simulink model "quad_sim"  (Simulink 6.2)
settings: Solver=ode45  StartTime=0.0  StopTime=70  MaxStep=0.001  RelTol=1e-3
libraries: aerospace x2

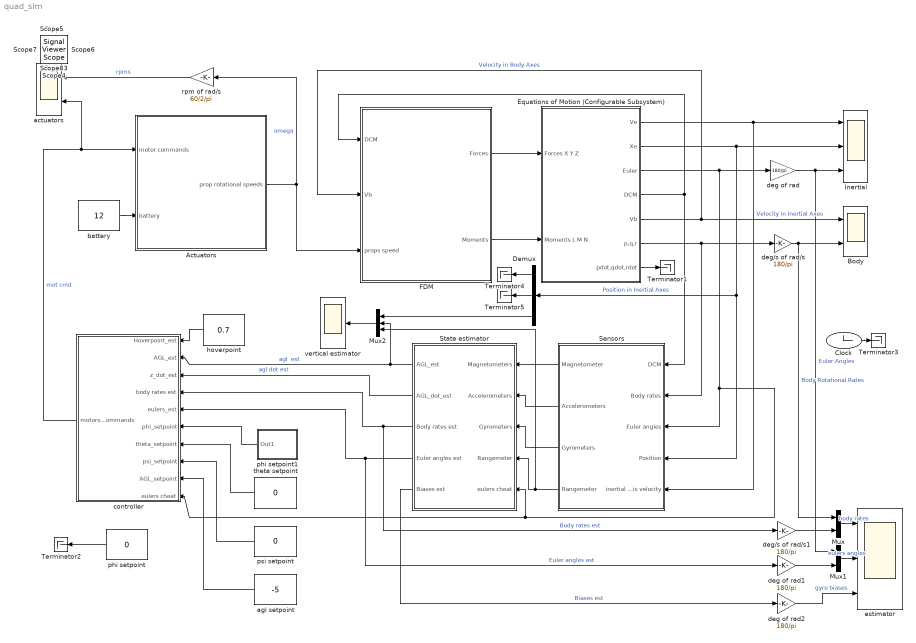
== system quad_sim ==
  Actuators : Subsystem  mask{Kv=1500, Tau=25, Kq=0.02}
  Body : Scope  NumInputPorts=2
  Clock : Clock
  Demux : Demux  Orientation=left  Outputs=3
  Equations of Motion (Configurable Subsystem) : Subsystem  BlockChoice=Euler Angles
      link override Euler Angles: Mass=0.5  Vm_0=[0 0 0]  Inertia=[0.0112 0 0; 0 0.0112 0; 0 0 0.0225]
  FDM : Subsystem  mask{Rho=1.225, Prop_area=0.005, Prop_radius=0.125, Mass=0.5, L=0.25, Ct=1.05, Cq=1.0, Cd_b=0.15}
      mask prompts: L "arm len"; Ct "Thrust aerodynamic coef"; Cq "Moment aerodynamic coef"; Cd_b "Body drag coef"
  Inertial : Scope  NumInputPorts=3
  Mux : Mux  Inputs=2
  Mux1 : Mux  Inputs=2
  Mux2 : Mux  Orientation=left  Inputs=3
  Sensors : Subsystem  Orientation=left
  State estimator : Subsystem  Orientation=left
  Terminator{1..5} (5 alike) : Terminator
  actuators : Scope  NumInputPorts=2
  agl setpoint : Constant  Orientation=left  Value=-5
  battery : Constant  Value=12
  controller : Subsystem  Orientation=left  mask{Kp_z=0.2, Kd_z=0.2, Kp_phi=-1.5, Kd_phi=-2.5, Kp_psi=-0.5, Kd_psi=-0.5}
  deg of rad : Gain  Gain=180/pi  SaturateOnIntegerOverflow=on
  deg of rad1 : Gain  Gain=180/pi  SaturateOnIntegerOverflow=on
  deg of rad2 : Gain  Gain=180/pi  SaturateOnIntegerOverflow=on
  deg/s of rad/s : Gain  Gain=180/pi  SaturateOnIntegerOverflow=on
  deg/s of rad/s1 : Gain  Gain=180/pi  SaturateOnIntegerOverflow=on
  estimator : Scope  NumInputPorts=3
  hoverpoint : Constant  Orientation=left  Value=0.7
  phi setpoint : Constant  Orientation=left  Value=0
  phi setpoint1 : Subsystem  Orientation=left  mask(timed input){t=[0 10 10 20 20 30 30 40 40 60], u=[0 0  -1 -1 0 0 1 1 0 0]*10/180*pi}
      mask prompts: t "time values:"; u "input values"
  psi setpoint : Constant  Orientation=left  Value=0
  rpm of rad/s : Gain  Orientation=left  Gain=60/2/pi  SaturateOnIntegerOverflow=on
  theta setpoint : Constant  Orientation=left  Value=0
  vertical estimator : Scope
  Scope{,1..8} (9 alike) : SignalViewerScope  IOType=viewer  RefreshTime=0.035000
  wires:
  Clock/1 -> Terminator3/1
  Equations of Motion (Configurable Subsystem)/3(Euler) -> deg of rad/1, Sensors/3(Euler angles), State estimator/5(eulers cheat), controller/10(eulers cheat)
  Equations of Motion (Configurable Subsystem)/5(Vb) -> Body/1, FDM/2(Vb)  "Velocity in Body Axes"
  Equations of Motion (Configurable Subsystem)/1(Ve) -> Inertial/1, Sensors/5(inertial axis velocity)  "Velocity in Inertial Axes"
  Equations of Motion (Configurable Subsystem)/2(Xe) -> Inertial/2, Sensors/4(Position), Demux/1  "Position in Inertial Axes"
  deg of rad/1 -> Inertial/3, Mux1/1  "Euler Angles"
  Equations of Motion (Configurable Subsystem)/6(p,q,r) -> deg/s of rad/s/1, Sensors/2(Body rates)
  deg/s of rad/s/1 -> Body/2, Mux/1  "Body Rotational Rates"
  Equations of Motion (Configurable Subsystem)/7(pdot,qdot,rdot) -> Terminator1/1
  FDM/2(Moments) -> Equations of Motion (Configurable Subsystem)/2(Moments L M N)
  FDM/1(Forces) -> Equations of Motion (Configurable Subsystem)/1(Forces X Y Z)
  Equations of Motion (Configurable Subsystem)/4(DCM) -> FDM/1(DCM), Sensors/1(DCM)
  battery/1 -> Actuators/2(battery)
  Actuators/1(prop rotational speeds) -> rpm of rad/s/1, FDM/3(props speed)  "omega"
  rpm of rad/s/1 -> actuators/1  "rpms"
  controller/1(motors commands) -> Actuators/1(motor commands), actuators/2  "mot cmd"
  hoverpoint/1 -> controller/1(Hoverpoint_est)
  agl setpoint/1 -> controller/9(AGL_setpoint)
  Sensors/4(Rangemeter) -> State estimator/4(Rangemeter), Mux2/3
  psi setpoint/1 -> controller/8(psi_setpoint)
  theta setpoint/1 -> controller/7(theta_setpoint)
  State estimator/3(Body rates est) -> controller/4(body rates est), deg/s of rad/s1/1  "Body rates est"
  State estimator/4(Euler angles est) -> controller/5(eulers_est), deg of rad1/1  "Euler angles est"
  Sensors/1(Magnetometer) -> State estimator/1(Magnetometers)
  Sensors/2(Accelerometers) -> State estimator/2(Accelerometers)
  Sensors/3(Gyrometers) -> State estimator/3(Gyrometers)
  Mux/1 -> estimator/1  "body rates"
  deg/s of rad/s1/1 -> Mux/2
  Mux1/1 -> estimator/2  "eulers angles"
  deg of rad1/1 -> Mux1/2
  phi setpoint1/1(Out1) -> controller/6(phi_setpoint)
  deg of rad2/1 -> estimator/3  "gyro biases"
  State estimator/5(Biases est) -> deg of rad2/1  "Biases est"
  phi setpoint/1 -> Terminator2/1
  Mux2/1 -> vertical estimator/1
  Demux/1 -> Terminator4/1
  Demux/2 -> Terminator5/1
  Demux/3 -> Mux2/1
  State estimator/1(AGL_est) -> controller/2(AGL_est), Mux2/2  "agl  est"
  State estimator/2(AGL_dot_est) -> controller/3(z_dot_est)  "agl dot est"

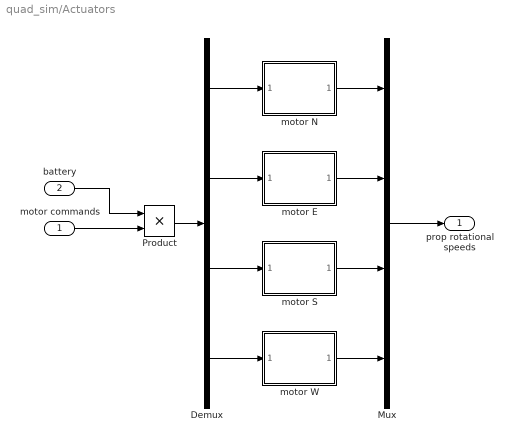
== system quad_sim/Actuators ==
  motor commands : Inport  Port=1  LatchInput=off
  battery : Inport  Port=2  LatchInput=off
  Demux : Demux
  Mux : Mux
  Product : Product  RndMeth=Zero
  motor E : Subsystem
  motor N : Subsystem
  motor S : Subsystem
  motor W : Subsystem
  prop rotational speeds : Outport
  wires:
  motor commands/1 -> Product/2
  battery/1 -> Product/1
  Product/1 -> Demux/1
  Mux/1 -> prop rotational speeds/1
  Demux/1 -> motor N/1(voltage)
  Demux/2 -> motor E/1(voltage)
  Demux/3 -> motor S/1(voltage)
  Demux/4 -> motor W/1(voltage)
  motor N/1(omega) -> Mux/1
  motor E/1(omega) -> Mux/2
  motor S/1(omega) -> Mux/3
  motor W/1(omega) -> Mux/4

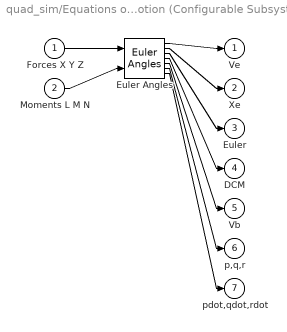
== system quad_sim/Equations of Motion (Configurable Subsystem) ==
  Forces X Y Z : Inport  Port=1  LatchInput=off
  Moments L M N : Inport  Port=2  LatchInput=off
  Euler Angles : aerospace/6DoF/Euler Angles  xme_0=[0 0 0]  Vm_0=[0 0 0]  eul_0=[0 0 0]  pm_0=[0 0 0]  Mass=0.5  Inertia=[0.0112 0 0; 0 0.0112 0; 0 0 0.0225]
  Ve : Outport
  Xe : Outport  Port=2
  Euler : Outport  Port=3
  DCM : Outport  Port=4
  Vb : Outport  Port=5
  p,q,r : Outport  Port=6
  pdot,qdot,rdot : Outport  Port=7
  wires:
  Forces X Y Z/1 -> Euler Angles/1
  Moments L M N/1 -> Euler Angles/2
  Euler Angles/1 -> Ve/1
  Euler Angles/2 -> Xe/1
  Euler Angles/3 -> Euler/1
  Euler Angles/4 -> DCM/1
  Euler Angles/5 -> Vb/1
  Euler Angles/6 -> p,q,r/1
  Euler Angles/7 -> pdot,qdot,rdot/1

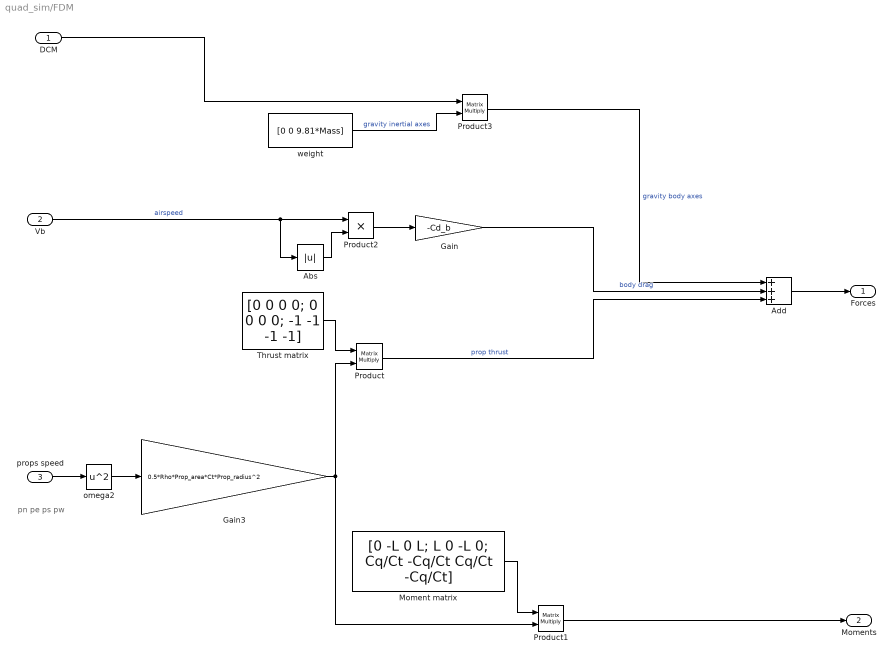
== system quad_sim/FDM ==
  note: pn
      | pe
      | ps
      | pw
  DCM : Inport  Port=1  LatchInput=off
  Vb : Inport  Port=2  LatchInput=off
  props speed : Inport  Port=3  LatchInput=off
  Abs : Abs
  Add : Sum  Inputs=+++  OutScaling=2^-10
  Gain : Gain  Gain=-Cd_b
  Gain3 : Gain  Gain=0.5*Rho*Prop_area*Ct*Prop_radius^2
  Moment matrix : Constant  Value=[0 -L 0 L; L 0 -L 0; Cq/Ct -Cq/Ct Cq/Ct -Cq/Ct]  VectorParams1D=off
  Product : Product  Multiplication=Matrix(*)  RndMeth=Zero
  Product1 : Product  Multiplication=Matrix(*)  RndMeth=Zero
  Product2 : Product  RndMeth=Zero
  Product3 : Product  Multiplication=Matrix(*)  RndMeth=Zero
  Thrust matrix : Constant  Value=[0 0 0 0; 0 0 0 0; -1 -1 -1 -1]  VectorParams1D=off
  omega2 : Math  Operator=square  SaturateOnIntegerOverflow=on
  weight : Constant  Value=[0 0 9.81*Mass]
  Forces : Outport
  Moments : Outport  Port=2
  wires:
  omega2/1 -> Gain3/1
  props speed/1 -> omega2/1
  Product1/1 -> Moments/1
  Add/1 -> Forces/1
  Product/1 -> Add/3  "prop thrust"
  Thrust matrix/1 -> Product/1
  Gain3/1 -> Product/2, Product1/2
  Moment matrix/1 -> Product1/1
  Vb/1 -> Abs/1, Product2/1  "airspeed"
  Product2/1 -> Gain/1
  Abs/1 -> Product2/2
  DCM/1 -> Product3/1
  Gain/1 -> Add/2  "body drag"
  weight/1 -> Product3/2  "gravity inertial axes"
  Product3/1 -> Add/1  "gravity body axes"

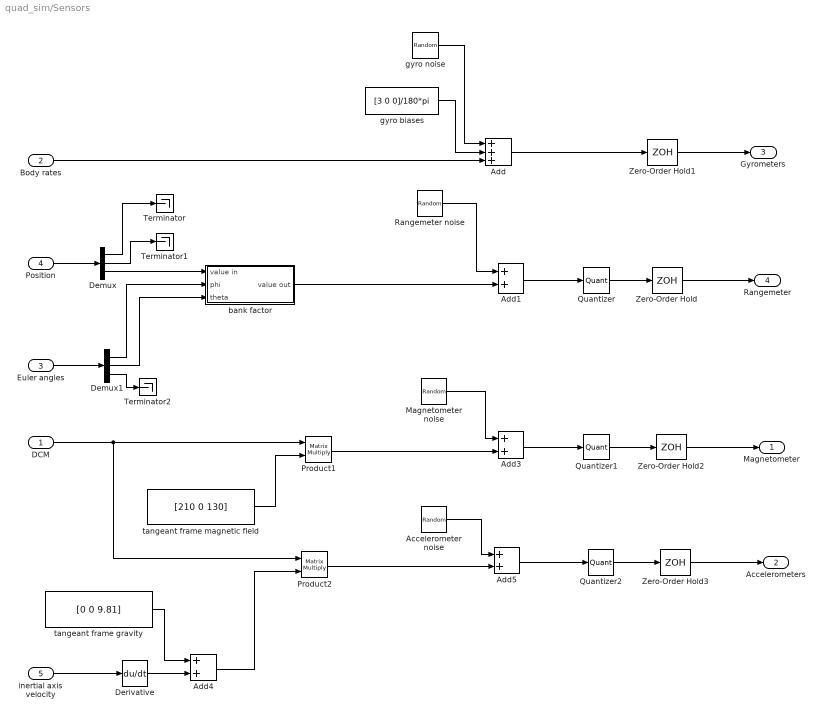
== system quad_sim/Sensors ==
  DCM : Inport  Port=1  LatchInput=off
  Body rates : Inport  Port=2  LatchInput=off
  Euler angles : Inport  Port=3  LatchInput=off
  Position : Inport  Port=4  LatchInput=off
  inertial axis velocity : Inport  Port=5  LatchInput=off
  Accelerometer noise : RandomNumber  Variance=0.001  SampleTime=0
  Add : Sum  Inputs=+++  OutScaling=2^-10
  Add{1,3..5} (4 alike) : Sum  OutScaling=2^-10
  Demux : Demux  Outputs=3
  Demux1 : Demux  Outputs=3
  Derivative : Derivative
  Magnetometer noise : RandomNumber  Variance=0.001  SampleTime=0
  Product1 : Product  Multiplication=Matrix(*)  RndMeth=Zero
  Product2 : Product  Multiplication=Matrix(*)  RndMeth=Zero
  Quantizer : Quantizer  QuantizationInterval=0.0254
  Quantizer1 : Quantizer  QuantizationInterval=1
  Quantizer2 : Quantizer  QuantizationInterval=0.1
  Rangemeter noise : RandomNumber  Variance=0.0025  SampleTime=0
  Terminator : Terminator
  Terminator1 : Terminator
  Terminator2 : Terminator
  Zero-Order Hold{,1..3} (4 alike) : ZeroOrderHold  SampleTime=0.016
  bank factor : Subsystem
  gyro biases : Constant  Value=[3 0 0]/180*pi
  gyro noise : RandomNumber  Mean=[0 0 0]  Variance=[0.0001 0.0001 0.0001]  SampleTime=0
  tangeant frame gravity : Constant  Value=[0 0 9.81]
  tangeant frame magnetic field : Constant  Value=[210 0 130]
  Magnetometer : Outport
  Accelerometers : Outport  Port=2
  Gyrometers : Outport  Port=3
  Rangemeter : Outport  Port=4
  wires:
  Body rates/1 -> Add/3
  gyro biases/1 -> Add/2
  gyro noise/1 -> Add/1
  Rangemeter noise/1 -> Add1/1
  Position/1 -> Demux/1
  Demux/1 -> Terminator/1
  Demux/2 -> Terminator1/1
  Zero-Order Hold/1 -> Rangemeter/1
  Quantizer/1 -> Zero-Order Hold/1
  Add1/1 -> Quantizer/1
  Zero-Order Hold1/1 -> Gyrometers/1
  Add/1 -> Zero-Order Hold1/1
  Euler angles/1 -> Demux1/1
  Demux1/3 -> Terminator2/1
  DCM/1 -> Product1/1, Product2/1
  tangeant frame magnetic field/1 -> Product1/2
  Product1/1 -> Add3/2
  Magnetometer noise/1 -> Add3/1
  Add3/1 -> Quantizer1/1
  Quantizer1/1 -> Zero-Order Hold2/1
  Zero-Order Hold2/1 -> Magnetometer/1
  inertial axis velocity/1 -> Derivative/1
  Derivative/1 -> Add4/2
  tangeant frame gravity/1 -> Add4/1
  Add4/1 -> Product2/2
  Quantizer2/1 -> Zero-Order Hold3/1
  Zero-Order Hold3/1 -> Accelerometers/1
  Product2/1 -> Add5/2
  Accelerometer noise/1 -> Add5/1
  Add5/1 -> Quantizer2/1
  Demux1/1 -> bank factor/2(phi)
  Demux1/2 -> bank factor/3(theta)
  Demux/3 -> bank factor/1(value in)
  bank factor/1(value out) -> Add1/2

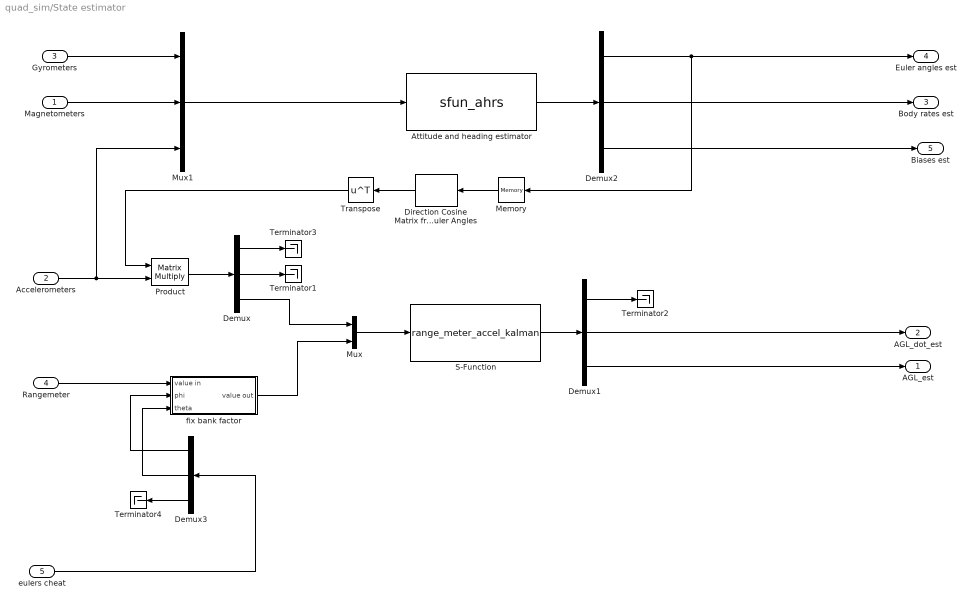
== system quad_sim/State estimator ==
  Magnetometers : Inport  Port=1  LatchInput=off
  Accelerometers : Inport  Port=2  LatchInput=off
  Gyrometers : Inport  Port=3  LatchInput=off
  Rangemeter : Inport  Port=4  LatchInput=off
  eulers cheat : Inport  Port=5  LatchInput=off
  Attitude and heading estimator : S-Function  FunctionName=sfun_ahrs
  Demux : Demux  Outputs=3
  Demux1 : Demux  Outputs=3
  Demux2 : Demux  Outputs=3
  Demux3 : Demux  Orientation=left  Outputs=3
  Direction Cosine Matrix from Euler Angles : aerospace/Axes Transformations/Direction Cosine Matrix from Euler Angles  Orientation=left
  Memory : Memory  Orientation=left
  Mux : Mux  Inputs=2
  Mux1 : Mux  Inputs=3
  Product : Product  Multiplication=Matrix(*)  SaturateOnIntegerOverflow=on  RndMeth=Zero  InputSameDT=on
  S-Function : S-Function  FunctionName=range_meter_accel_kalman
  Terminator{1..4} (4 alike) : Terminator
  Transpose : Math  Orientation=left  Operator=transpose  SaturateOnIntegerOverflow=on
  fix bank factor : Subsystem
  AGL_est : Outport
  AGL_dot_est : Outport  Port=2
  Body rates est : Outport  Port=3
  Euler angles est : Outport  Port=4
  Biases est : Outport  Port=5
  wires:
  Accelerometers/1 -> Mux1/3, Product/2
  Demux/1 -> Terminator3/1
  Demux/2 -> Terminator1/1
  Demux/3 -> Mux/1
  Mux/1 -> S-Function/1
  S-Function/1 -> Demux1/1
  Demux1/1 -> Terminator2/1
  Demux1/2 -> AGL_dot_est/1
  Demux1/3 -> AGL_est/1
  Gyrometers/1 -> Mux1/1
  Magnetometers/1 -> Mux1/2
  Mux1/1 -> Attitude and heading estimator/1
  Attitude and heading estimator/1 -> Demux2/1
  Demux2/1 -> Euler angles est/1, Memory/1
  Demux2/2 -> Body rates est/1
  Demux2/3 -> Biases est/1
  Memory/1 -> Direction Cosine Matrix from Euler Angles/1
  Direction Cosine Matrix from Euler Angles/1 -> Transpose/1
  Product/1 -> Demux/1
  Transpose/1 -> Product/1
  Rangemeter/1 -> fix bank factor/1(value in)
  fix bank factor/1(value out) -> Mux/2
  Demux3/1 -> fix bank factor/2(phi)
  Demux3/2 -> fix bank factor/3(theta)
  Demux3/3 -> Terminator4/1
  eulers cheat/1 -> Demux3/1

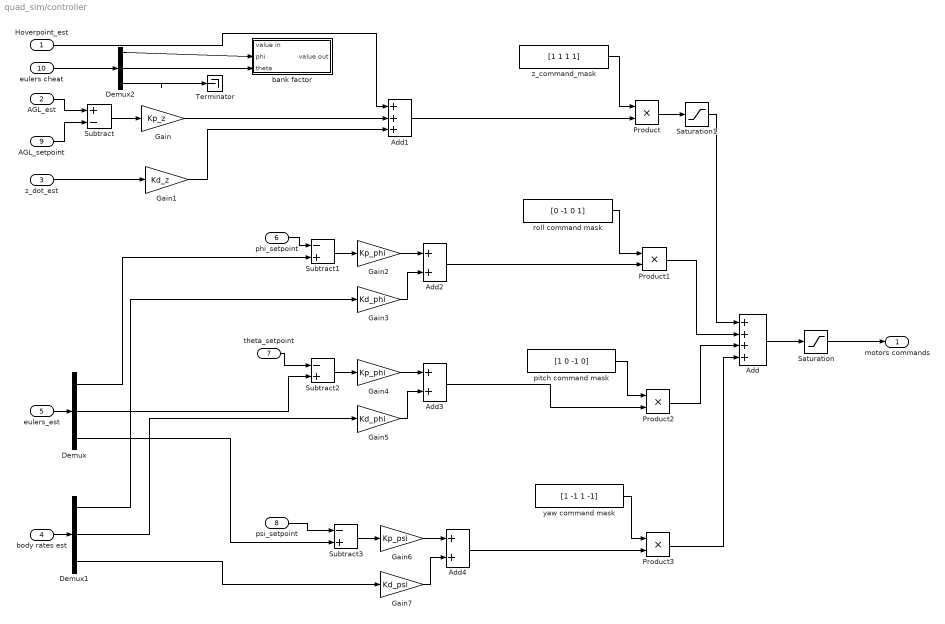
== system quad_sim/controller ==
  Hoverpoint_est : Inport  Port=1  LatchInput=off
  AGL_est : Inport  Port=2  LatchInput=off
  z_dot_est : Inport  Port=3  LatchInput=off
  body rates est : Inport  Port=4  LatchInput=off
  eulers_est : Inport  Port=5  LatchInput=off
  phi_setpoint : Inport  Port=6  LatchInput=off
  theta_setpoint : Inport  Port=7  LatchInput=off
  psi_setpoint : Inport  Port=8  LatchInput=off
  AGL_setpoint : Inport  Port=9  LatchInput=off
  eulers cheat : Inport  Port=10  LatchInput=off
  Add : Sum  Inputs=++++  OutScaling=2^-10
  Add1 : Sum  Inputs=+++  OutScaling=2^-10
  Add2 : Sum  OutScaling=2^-10
  Add3 : Sum  OutScaling=2^-10
  Add4 : Sum  OutScaling=2^-10
  Demux : Demux  Outputs=3
  Demux1 : Demux  Outputs=3
  Demux2 : Demux  Outputs=3
  Gain : Gain  Gain=Kp_z
  Gain1 : Gain  Gain=Kd_z
  Gain2 : Gain  Gain=Kp_phi
  Gain3 : Gain  Gain=Kd_phi
  Gain4 : Gain  Gain=Kp_phi
  Gain5 : Gain  Gain=Kd_phi
  Gain6 : Gain  Gain=Kp_psi
  Gain7 : Gain  Gain=Kd_psi
  Product{,1..3} (4 alike) : Product  RndMeth=Zero
  Saturation : Saturate  UpperLimit=[1 1 1 1]  LowerLimit=[0 0 0 0]
  Saturation1 : Saturate  UpperLimit=[1 1 1 1]*0.9  LowerLimit=[0 0 0 0]
  Subtract : Sum  Inputs=+-  OutScaling=2^-10
  Subtract1 : Sum  Inputs=-+  OutScaling=2^-10
  Subtract2 : Sum  Inputs=-+  OutScaling=2^-10
  Subtract3 : Sum  Inputs=-+  OutScaling=2^-10
  Terminator : Terminator
  bank factor : Subsystem
  pitch command mask : Constant  Value=[1 0 -1 0]
  roll command mask : Constant  Value=[0 -1 0 1]
  yaw command mask : Constant  Value=[1 -1 1 -1]
  z_command_mask : Constant  Value=[1 1 1 1]
  motors commands : Outport
  wires:
  AGL_est/1 -> Subtract/1
  AGL_setpoint/1 -> Subtract/2
  Subtract/1 -> Gain/1
  Gain/1 -> Add1/2
  Add1/1 -> Product/2
  z_command_mask/1 -> Product/1
  roll command mask/1 -> Product1/1
  Add2/1 -> Product1/2
  Product1/1 -> Add/2
  pitch command mask/1 -> Product2/1
  Add3/1 -> Product2/2
  Product2/1 -> Add/3
  yaw command mask/1 -> Product3/1
  Add4/1 -> Product3/2
  Product3/1 -> Add/4
  z_dot_est/1 -> Gain1/1
  Gain1/1 -> Add1/3
  Add/1 -> Saturation/1
  Saturation/1 -> motors commands/1
  eulers_est/1 -> Demux/1
  body rates est/1 -> Demux1/1
  phi_setpoint/1 -> Subtract1/1
  Demux/1 -> Subtract1/2
  Subtract1/1 -> Gain2/1
  Gain2/1 -> Add2/1
  Gain3/1 -> Add2/2
  Demux1/1 -> Gain3/1
  Subtract2/1 -> Gain4/1
  Gain4/1 -> Add3/1
  Gain5/1 -> Add3/2
  theta_setpoint/1 -> Subtract2/1
  Demux/2 -> Subtract2/2
  Demux1/2 -> Gain5/1
  Subtract3/1 -> Gain6/1
  Gain6/1 -> Add4/1
  Gain7/1 -> Add4/2
  psi_setpoint/1 -> Subtract3/1
  Demux/3 -> Subtract3/2
  Demux1/3 -> Gain7/1
  Product/1 -> Saturation1/1
  Saturation1/1 -> Add/1
  eulers cheat/1 -> Demux2/1
  Demux2/1 -> bank factor/2(phi)
  Demux2/2 -> bank factor/3(theta)
  Demux2/3 -> Terminator/1
  Hoverpoint_est/1 -> Add1/1

== system quad_sim/phi setpoint1 ==
  From  Workspace : FromWorkspace  VariableName=[t',u']  SampleTime=0
  Out1 : Outport  InitialOutput=0
  wires:
  From  Workspace/1 -> Out1/1

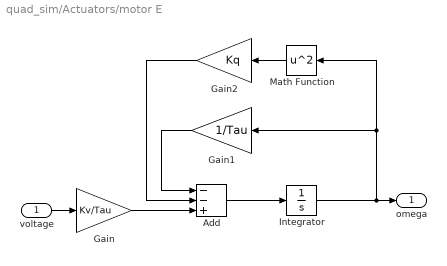
== system quad_sim/Actuators/motor E ==
  voltage : Inport  Port=1  LatchInput=off
  Add : Sum  Inputs=--+  OutScaling=2^-10
  Gain : Gain  Gain=Kv/Tau
  Gain1 : Gain  Orientation=left  Gain=1/Tau
  Gain2 : Gain  Orientation=left  Gain=Kq
  Integrator : Integrator
  Math Function : Math  Orientation=left  Operator=square  SaturateOnIntegerOverflow=on
  omega : Outport
  wires:
  Gain/1 -> Add/3
  Add/1 -> Integrator/1
  Integrator/1 -> Math Function/1, Gain1/1, omega/1
  Math Function/1 -> Gain2/1
  Gain2/1 -> Add/2
  Gain1/1 -> Add/1
  voltage/1 -> Gain/1

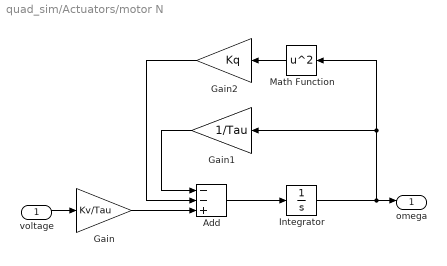
== system quad_sim/Actuators/motor N ==
  voltage : Inport  Port=1  LatchInput=off
  Add : Sum  Inputs=--+  OutScaling=2^-10
  Gain : Gain  Gain=Kv/Tau
  Gain1 : Gain  Orientation=left  Gain=1/Tau
  Gain2 : Gain  Orientation=left  Gain=Kq
  Integrator : Integrator
  Math Function : Math  Orientation=left  Operator=square  SaturateOnIntegerOverflow=on
  omega : Outport
  wires:
  Gain/1 -> Add/3
  Add/1 -> Integrator/1
  Integrator/1 -> Math Function/1, Gain1/1, omega/1
  Math Function/1 -> Gain2/1
  Gain2/1 -> Add/2
  Gain1/1 -> Add/1
  voltage/1 -> Gain/1

== system quad_sim/Actuators/motor S ==
  voltage : Inport  Port=1  LatchInput=off
  Add : Sum  Inputs=--+  OutScaling=2^-10
  Gain : Gain  Gain=Kv/Tau
  Gain1 : Gain  Orientation=left  Gain=1/Tau
  Gain2 : Gain  Orientation=left  Gain=Kq
  Integrator : Integrator
  Math Function : Math  Orientation=left  Operator=square  SaturateOnIntegerOverflow=on
  omega : Outport
  wires:
  Gain/1 -> Add/3
  Add/1 -> Integrator/1
  Integrator/1 -> Math Function/1, Gain1/1, omega/1
  Math Function/1 -> Gain2/1
  Gain2/1 -> Add/2
  Gain1/1 -> Add/1
  voltage/1 -> Gain/1

== system quad_sim/Actuators/motor W ==
  voltage : Inport  Port=1  LatchInput=off
  Add : Sum  Inputs=--+  OutScaling=2^-10
  Gain : Gain  Gain=Kv/Tau
  Gain1 : Gain  Orientation=left  Gain=1/Tau
  Gain2 : Gain  Orientation=left  Gain=Kq
  Integrator : Integrator
  Math Function : Math  Orientation=left  Operator=square  SaturateOnIntegerOverflow=on
  omega : Outport
  wires:
  Gain/1 -> Add/3
  Add/1 -> Integrator/1
  Integrator/1 -> Math Function/1, Gain1/1, omega/1
  Math Function/1 -> Gain2/1
  Gain2/1 -> Add/2
  Gain1/1 -> Add/1
  voltage/1 -> Gain/1

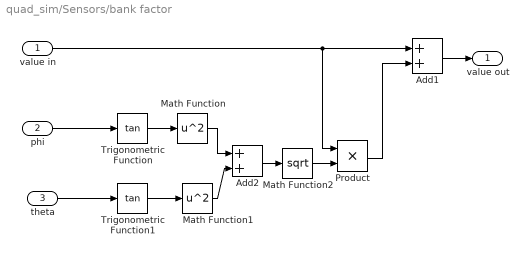
== system quad_sim/Sensors/bank factor ==
  value in : Inport  Port=1  LatchInput=off
  phi : Inport  Port=2  LatchInput=off
  theta : Inport  Port=3  LatchInput=off
  Add1 : Sum  OutScaling=2^-10
  Add2 : Sum  OutScaling=2^-10
  Math Function : Math  Operator=square  SaturateOnIntegerOverflow=on
  Math Function1 : Math  Operator=square  SaturateOnIntegerOverflow=on
  Math Function2 : Math  Operator=sqrt  SaturateOnIntegerOverflow=on
  Product : Product  RndMeth=Zero
  Trigonometric Function : Trigonometry  Operator=tan
  Trigonometric Function1 : Trigonometry  Operator=tan
  value out : Outport
  wires:
  Trigonometric Function1/1 -> Math Function1/1
  Trigonometric Function/1 -> Math Function/1
  Math Function/1 -> Add2/1
  Math Function1/1 -> Add2/2
  Add2/1 -> Math Function2/1
  Math Function2/1 -> Product/2
  theta/1 -> Trigonometric Function1/1
  phi/1 -> Trigonometric Function/1
  value in/1 -> Add1/1, Product/1
  Add1/1 -> value out/1
  Product/1 -> Add1/2

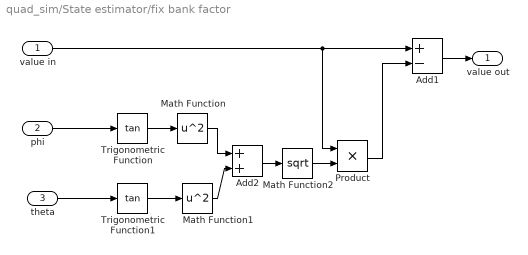
== system quad_sim/State estimator/fix bank factor ==
  value in : Inport  Port=1  LatchInput=off
  phi : Inport  Port=2  LatchInput=off
  theta : Inport  Port=3  LatchInput=off
  Add1 : Sum  Inputs=+-  OutScaling=2^-10
  Add2 : Sum  OutScaling=2^-10
  Math Function : Math  Operator=square  SaturateOnIntegerOverflow=on
  Math Function1 : Math  Operator=square  SaturateOnIntegerOverflow=on
  Math Function2 : Math  Operator=sqrt  SaturateOnIntegerOverflow=on
  Product : Product  RndMeth=Zero
  Trigonometric Function : Trigonometry  Operator=tan
  Trigonometric Function1 : Trigonometry  Operator=tan
  value out : Outport
  wires:
  Trigonometric Function1/1 -> Math Function1/1
  Trigonometric Function/1 -> Math Function/1
  Math Function/1 -> Add2/1
  Math Function1/1 -> Add2/2
  Add2/1 -> Math Function2/1
  Math Function2/1 -> Product/2
  theta/1 -> Trigonometric Function1/1
  phi/1 -> Trigonometric Function/1
  value in/1 -> Add1/1, Product/1
  Add1/1 -> value out/1
  Product/1 -> Add1/2

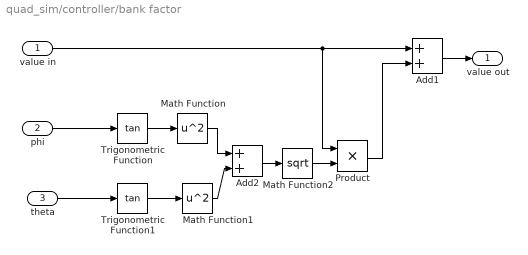
== system quad_sim/controller/bank factor ==
  value in : Inport  Port=1  LatchInput=off
  phi : Inport  Port=2  LatchInput=off
  theta : Inport  Port=3  LatchInput=off
  Add1 : Sum  OutScaling=2^-10
  Add2 : Sum  OutScaling=2^-10
  Math Function : Math  Operator=square  SaturateOnIntegerOverflow=on
  Math Function1 : Math  Operator=square  SaturateOnIntegerOverflow=on
  Math Function2 : Math  Operator=sqrt  SaturateOnIntegerOverflow=on
  Product : Product  RndMeth=Zero
  Trigonometric Function : Trigonometry  Operator=tan
  Trigonometric Function1 : Trigonometry  Operator=tan
  value out : Outport
  wires:
  Trigonometric Function1/1 -> Math Function1/1
  Trigonometric Function/1 -> Math Function/1
  Math Function/1 -> Add2/1
  Math Function1/1 -> Add2/2
  Add2/1 -> Math Function2/1
  Math Function2/1 -> Product/2
  theta/1 -> Trigonometric Function1/1
  phi/1 -> Trigonometric Function/1
  value in/1 -> Add1/1, Product/1
  Add1/1 -> value out/1
  Product/1 -> Add1/2
